simulink model "HEVModel"  (R2021a)
settings: Solver=ode4  StartTime=0  StopTime=tEnd  FixedStep=dt  RelTol=1e-3
values from neighbouring files (symbols this model uses):
  accessoryLoad = 600    [main.m]
  Af = 1.00    (= 1)    [main.m]
  batteryCapacity = 50    [main.m]
  batteryResistance = 0.0461    [main.m]
  C = 400    [main.m]
  Cd = 0.576    [main.m]
  Crr = 0.01    [main.m]
  cycleNum = 2    [main.m]
  EffTableEff = [.75 .85 .89 .95 .96 .97 .98 .99 .99]    [main.m]
  EffTableSpeed = [0 5 10 15 25 35 45 55 65]    [main.m]
  etaGenGR = 0.93    [main.m]
  g = 9.81    [main.m]
  genMotorData = load(GENERATOR_MOTOR_DATA_NAME)    [main.m]
  GRd = 9.843    [main.m]
  GRgen = 1.4    [main.m]
  initialGasVolume = 5    [main.m]
  k_gal2kWh = 32.3    [main.m]
  k_hr2s = 3600    [main.m]
  k_J2gal = 1/3600000/32.3    (= 8.59993120055e-09)    [main.m]
  k_kW2W = 1000    [main.m]
  k_kWh2J = 3.6*10^6    (= 3600000)    [main.m]
  k_m2mi = 0.000621371    [main.m]
  k_m32gal = 264.172    [main.m]
  k_rpm2rps = 2*pi()/60    [main.m]
  k_rps2rpm = 60/(2*pi)    (= 9.54929658551)    [main.m]
  k_s2h = 1/3600    (= 0.000277777777778)    [main.m]
  k_W2kW = 1/1000    (= 0.001)    [main.m]
  kc = 0.513    [main.m]
  Kd = 0    [main.m]
  Ki = 0.1    [main.m]
  ki = 0.0773    [main.m]
  Kp = 200    [main.m]
  kw = 0.0000064    (= 6.4e-06)    [main.m]
  m = 1965    [main.m]
  motorMaxPower = 310000    [main.m]
  motorMaxSpeed = 18000    [main.m]
  motorMaxTorque = 600    [main.m]
  openCircuitVoltage = 420    [main.m]
  pBrakeMax = 4*TbrakeMax / (mu_k*pi()* cylinderBore^2 *meanPadRadius*numPads)    [main.m]
  r = 0.290    (= 0.29)    [main.m]
  rho = 1.20    (= 1.2)    [main.m]
  SOCi = 90    [main.m]
  theta = 0    [main.m]
  v0 = 0    [main.m]
  x0 = 0    [main.m]
libraries: autolibshared x6, fl_lib x5, nesl_utility x5, sdl_lib x1, autolibsharedmappedengines x1
(part 3 of 3)

== system HEVModel/Plant/Genset/Gearbox ==
  Torque In [Nm] : Inport
  Power In [W] : Inport  Port=2
  Engine Speed [rad/s] : Inport  Port=3
  Add : Sum  Inputs=+-
  Bus Creator : BusCreator  Inputs=3
  Gain : Gain  Gain=GRgen
  Gain1 : Gain  Gain=k_W2kW
  Gain2 : Gain  Gain=etaGenGR
  Gain3 : Gain  Gain=1/GRgen
  Product1 : Product
  Torque Out [Nm] : Outport
  Info : Outport  Port=2
  wires:
  Gain2/1 -> [torqueOut], Torque Out [Nm]/1, Product1/1  "Torque Out [Nm]"
  Product1/1 -> Add/2  "Gearbox Power Out [W]"
  Engine Speed [rad/s]/1 -> Gain3/1
  Gain/1 -> Gain2/1
  Power In [W]/1 -> Add/1
  Add/1 -> Gain1/1  "Gearbox Power Loss [W]"
  Torque In [Nm]/1 -> [torqueIn], Gain/1
  Gain1/1 -> Bus Creator/1  "powerLoss"
  [torqueIn] -> Bus Creator/2  "torqueIn"
  [torqueOut] -> Bus Creator/3  "torqueOut"
  Bus Creator/1 -> Info/1  "gearbox"
  Gain3/1 -> Product1/2

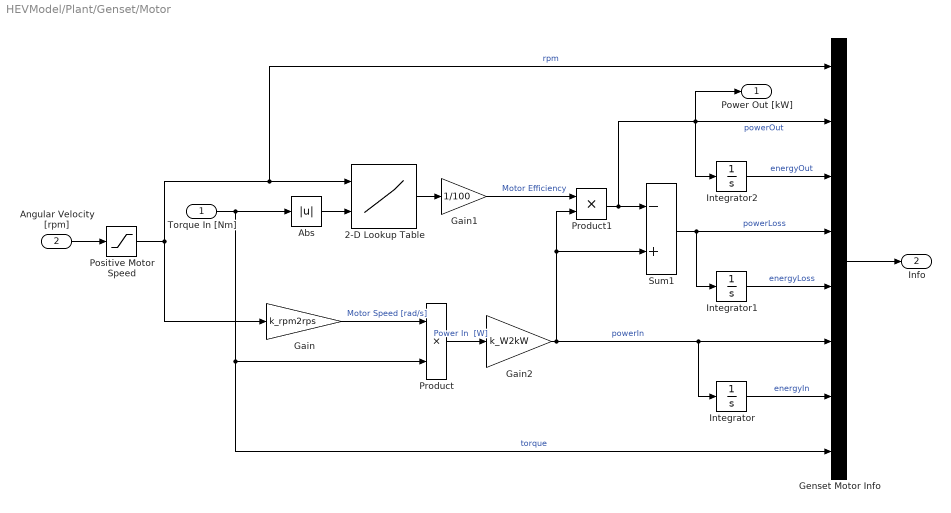
== system HEVModel/Plant/Genset/Motor ==
  Torque In [Nm] : Inport
  Angular Velocity [rpm] : Inport  Port=2
  2-D Lookup Table : Lookup_n-D  BreakpointsForDimension1=genMotorData.w_eff_bp  BreakpointsForDimension2=genMotorData.T_eff_bp  Table=genMotorData.efficiency_table  InternalRulePriority=Speed  RndMeth=Simplest  InputSameDT=on
      settings: InputPortMap=u0,u1
  Abs : Abs
  Gain : Gain  Gain=k_rpm2rps
  Gain1 : Gain  Gain=1/100
  Gain2 : Gain  Gain=k_W2kW
  Genset Motor Info : BusCreator  Inputs=8
  Integrator : Integrator
  Integrator1 : Integrator
  Integrator2 : Integrator
  Positive Motor Speed : Saturate  UpperLimit=inf  LowerLimit=0
  Product : Product
  Product1 : Product
  Sum1 : Sum  Inputs=-+
  Power Out [kW] : Outport
  Info : Outport  Port=2
  wires:
  Angular Velocity [rpm]/1 -> Positive Motor Speed/1
  Gain/1 -> Product/1  "Motor Speed [rad/s]"
  Positive Motor Speed/1 -> Genset Motor Info/1, 2-D Lookup Table/1, Gain/1  "rpm"
  Gain1/1 -> Product1/1  "Motor Efficiency"
  Product1/1 -> Sum1/1, Power Out [kW]/1, Genset Motor Info/2, Integrator2/1  "powerOut"
  Integrator2/1 -> Genset Motor Info/3  "energyOut"
  Sum1/1 -> Genset Motor Info/4, Integrator1/1  "powerLoss"
  2-D Lookup Table/1 -> Gain1/1
  Abs/1 -> 2-D Lookup Table/2
  Integrator1/1 -> Genset Motor Info/5  "energyLoss"
  Integrator/1 -> Genset Motor Info/7  "energyIn"
  Torque In [Nm]/1 -> Abs/1, Genset Motor Info/8, Product/2  "torque"
  Gain2/1 -> Integrator/1, Genset Motor Info/6, Sum1/2, Product1/2  "powerIn"
  Genset Motor Info/1 -> Info/1
  Product/1 -> Gain2/1  "Power In  [W]"

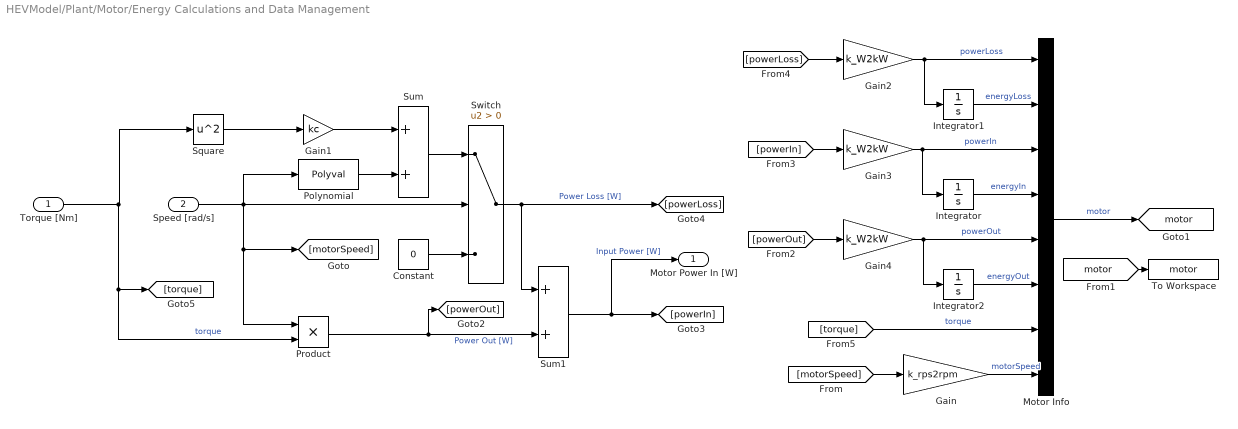
== system HEVModel/Plant/Motor/Energy Calculations and Data Management ==
  Torque [Nm] : Inport
  Speed [rad/s] : Inport  Port=2
  Constant : Constant  Value=0
  Gain : Gain  Gain=k_rps2rpm
  Gain1 : Gain  Gain=kc
  Gain2 : Gain  Gain=k_W2kW
  Gain3 : Gain  Gain=k_W2kW
  Gain4 : Gain  Gain=k_W2kW
  Integrator : Integrator
  Integrator1 : Integrator
  Integrator2 : Integrator
  Motor Info : BusCreator  Inputs=8
  Polynomial : Polyval  Coefs=[kw , 0 ki, C]
  Product : Product
  Square : Math  Operator=square  SaturateOnIntegerOverflow=on
  Sum : Sum
  Sum1 : Sum
  Switch : Switch  Criteria=u2 > Threshold
  To Workspace : ToWorkspace  VariableName=motor  SaveFormat=Timeseries  SampleTime=-1
  Motor Power In [W] : Outport
  tag scope: motor=global
  wires:
  Motor Info/1 -> [motor]  "motor"
  Product/1 -> [powerOut], Sum1/2  "Power Out [W]"
  Speed [rad/s]/1 -> Polynomial/1, Product/1, [motorSpeed], Switch/2
  Constant/1 -> Switch/3
  Polynomial/1 -> Sum/2
  Sum/1 -> Switch/1
  Gain1/1 -> Sum/1
  Switch/1 -> Sum1/1, [powerLoss]  "Power Loss [W]"
  Sum1/1 -> Motor Power In [W]/1, [powerIn]  "Input Power [W]"
  Torque [Nm]/1 -> Square/1, Product/2, [torque]  "torque"
  Square/1 -> Gain1/1
  Integrator/1 -> Motor Info/4  "energyIn"
  Integrator2/1 -> Motor Info/6  "energyOut"
  Integrator1/1 -> Motor Info/2  "energyLoss"
  [motorSpeed] -> Gain/1
  Gain/1 -> Motor Info/8  "motorSpeed"
  [motor] -> To Workspace/1
  Gain4/1 -> Integrator2/1, Motor Info/5  "powerOut"
  Gain3/1 -> Motor Info/3, Integrator/1  "powerIn"
  Gain2/1 -> Motor Info/1, Integrator1/1  "powerLoss"
  [torque] -> Motor Info/7  "torque"
  [powerLoss] -> Gain2/1
  [powerIn] -> Gain3/1
  [powerOut] -> Gain4/1

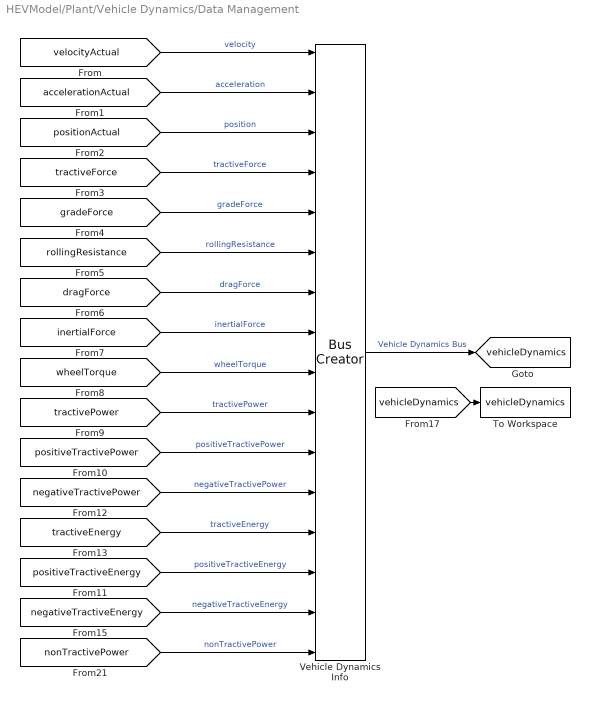
== system HEVModel/Plant/Vehicle Dynamics/Data Management ==
  To Workspace : ToWorkspace  VariableName=vehicleDynamics  SaveFormat=Timeseries  SampleTime=-1
  Vehicle Dynamics Info : BusCreator  Inputs=16
  tag scope: vehicleDynamics=global
  wires:
  [velocityActual] -> Vehicle Dynamics Info/1  "velocity"
  [wheelTorque] -> Vehicle Dynamics Info/9  "wheelTorque"
  [tractiveForce] -> Vehicle Dynamics Info/4  "tractiveForce"
  [negativeTractivePower] -> Vehicle Dynamics Info/12  "negativeTractivePower"
  [accelerationActual] -> Vehicle Dynamics Info/2  "acceleration"
  [vehicleDynamics] -> To Workspace/1
  [gradeForce] -> Vehicle Dynamics Info/5  "gradeForce"
  [positiveTractivePower] -> Vehicle Dynamics Info/11  "positiveTractivePower"
  [positiveTractiveEnergy] -> Vehicle Dynamics Info/14  "positiveTractiveEnergy"
  [rollingResistance] -> Vehicle Dynamics Info/6  "rollingResistance"
  [inertialForce] -> Vehicle Dynamics Info/8  "inertialForce"
  [positionActual] -> Vehicle Dynamics Info/3  "position"
  [tractivePower] -> Vehicle Dynamics Info/10  "tractivePower"
  [negativeTractiveEnergy] -> Vehicle Dynamics Info/15  "negativeTractiveEnergy"
  [tractiveEnergy] -> Vehicle Dynamics Info/13  "tractiveEnergy"
  [dragForce] -> Vehicle Dynamics Info/7  "dragForce"
  [nonTractivePower] -> Vehicle Dynamics Info/16  "nonTractivePower"
  Vehicle Dynamics Info/1 -> [vehicleDynamics]  "Vehicle Dynamics Bus"

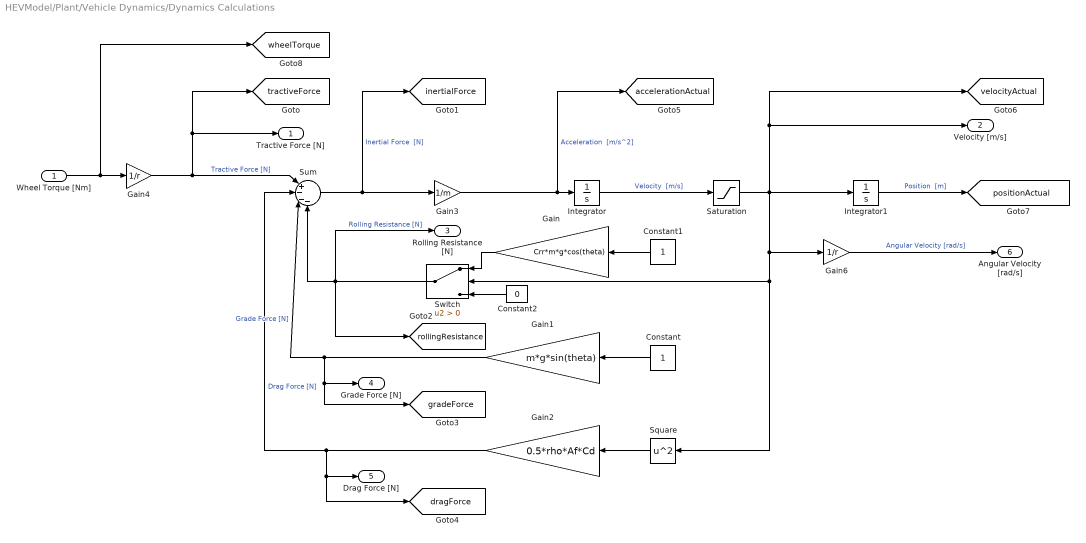
== system HEVModel/Plant/Vehicle Dynamics/Dynamics Calculations ==
  Wheel Torque [Nm] : Inport
  Constant : Constant
  Constant1 : Constant
  Constant2 : Constant  Value=0
  Gain : Gain  Gain=Crr*m*g*cos(theta)
  Gain1 : Gain  Gain=m*g*sin(theta)
  Gain2 : Gain  Gain=0.5*rho*Af*Cd
  Gain3 : Gain  Gain=1/m
  Gain4 : Gain  Gain=1/r
  Gain6 : Gain  Gain=1/r
  Integrator : Integrator  InitialCondition=v0
  Integrator1 : Integrator  InitialCondition=x0
  Saturation : Saturate  UpperLimit=inf  LowerLimit=0  LinearizeAsGain=off
  Square : Math  Operator=square  SaturateOnIntegerOverflow=on
  Sum : Sum  Inputs=|+---
  Switch : Switch  Criteria=u2 > Threshold
  Tractive Force [N] : Outport
  Velocity [m/s] : Outport  Port=2
  Rolling Resistance [N] : Outport  Port=3
  Grade Force [N] : Outport  Port=4
  Drag Force [N] : Outport  Port=5
  Angular Velocity [rad/s] : Outport  Port=6
  tag scope: accelerationActual=global, dragForce=global, gradeForce=global, inertialForce=global, positionActual=global, rollingResistance=global, tractiveForce=global, velocityActual=global, wheelTorque=global
  wires:
  Gain1/1 -> Grade Force [N]/1, [gradeForce], Sum/3  "Grade Force [N]"
  Gain4/1 -> Tractive Force [N]/1, [tractiveForce], Sum/1  "Tractive Force [N]"
  Constant/1 -> Gain1/1
  Switch/1 -> Sum/4, [rollingResistance], Rolling Resistance [N]/1  "Rolling Resistance [N]"
  Integrator/1 -> Saturation/1  "Velocity  [m/s]"
  Integrator1/1 -> [positionActual]  "Position  [m]"
  Sum/1 -> [inertialForce], Gain3/1  "Inertial Force  [N]"
  Constant1/1 -> Gain/1
  Gain3/1 -> [accelerationActual], Integrator/1  "Acceleration  [m/s^2]"
  Gain2/1 -> Drag Force [N]/1, [dragForce], Sum/2  "Drag Force [N]"
  Wheel Torque [Nm]/1 -> [wheelTorque], Gain4/1
  Square/1 -> Gain2/1
  Saturation/1 -> Gain6/1, Square/1, Switch/2, Velocity [m/s]/1, [velocityActual], Integrator1/1
  Gain/1 -> Switch/1
  Constant2/1 -> Switch/3
  Gain6/1 -> Angular Velocity [rad/s]/1  "Angular Velocity [rad/s]"

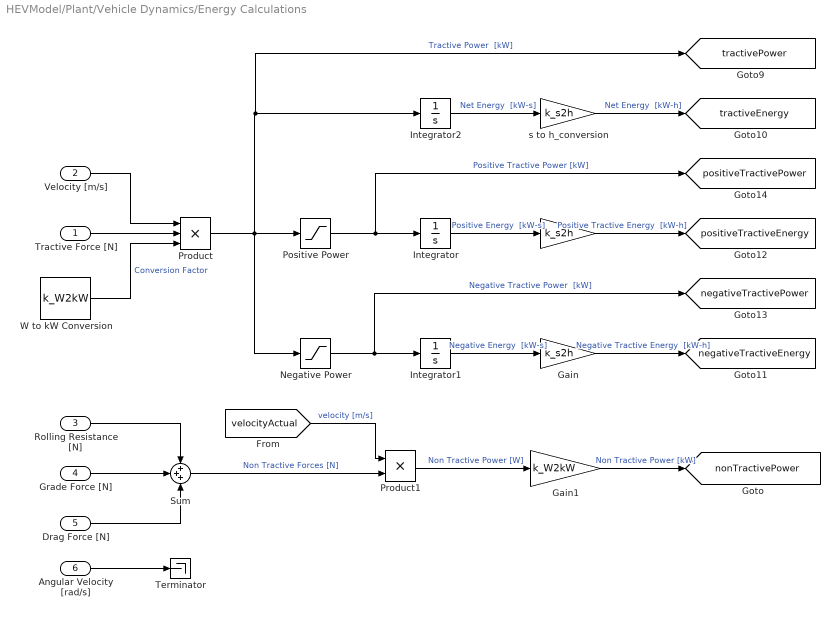
== system HEVModel/Plant/Vehicle Dynamics/Energy Calculations ==
  Tractive Force [N] : Inport
  Velocity [m/s] : Inport  Port=2
  Rolling Resistance [N] : Inport  Port=3
  Grade Force [N] : Inport  Port=4
  Drag Force [N] : Inport  Port=5
  Angular Velocity [rad/s] : Inport  Port=6
  " " : Gain  Gain=k_s2h
  Gain : Gain  Gain=k_s2h
  Gain1 : Gain  Gain=k_W2kW
  Integrator : Integrator
  Integrator1 : Integrator
  Integrator2 : Integrator
  Negative Power : Saturate  UpperLimit=0  LowerLimit=-inf
  Positive Power : Saturate  UpperLimit=inf  LowerLimit=0
  Product : Product  Inputs=3
  Product1 : Product
  Sum : Sum  Inputs=+++
  Terminator : Terminator
  W to kW Conversion : Constant  Value=k_W2kW
  s to h_conversion : Gain  Gain=k_s2h
  tag scope: negativeTractiveEnergy=global, negativeTractivePower=global, nonTractivePower=global, positiveTractiveEnergy=global, positiveTractivePower=global, tractiveEnergy=global, tractivePower=global
  wires:
  s to h_conversion/1 -> [tractiveEnergy]  "Net Energy  [kW-h]"
  " "/1 -> [positiveTractiveEnergy]  "Positive Tractive Energy  [kW-h]"
  Gain/1 -> [negativeTractiveEnergy]  "Negative Tractive Energy  [kW-h]"
  Integrator1/1 -> Gain/1  "Negative Energy  [kW-s]"
  Integrator/1 -> " "/1  "Positive Energy  [kW-s]"
  Negative Power/1 -> [negativeTractivePower], Integrator1/1  "Negative Tractive Power  [kW]"
  Integrator2/1 -> s to h_conversion/1  "Net Energy  [kW-s]"
  Positive Power/1 -> [positiveTractivePower], Integrator/1  "Positive Tractive Power [kW]"
  W to kW Conversion/1 -> Product/3  "Conversion Factor"
  Product/1 -> Negative Power/1, [tractivePower], Integrator2/1, Positive Power/1  "Tractive Power  [kW]"
  Velocity [m/s]/1 -> Product/1
  Tractive Force [N]/1 -> Product/2
  Drag Force [N]/1 -> Sum/3
  Grade Force [N]/1 -> Sum/2
  Rolling Resistance [N]/1 -> Sum/1
  Sum/1 -> Product1/2  "Non Tractive Forces [N]"
  [velocityActual] -> Product1/1  "velocity [m/s]"
  Product1/1 -> Gain1/1  "Non Tractive Power [W]"
  Gain1/1 -> [nonTractivePower]  "Non Tractive Power [kW]"
  Angular Velocity [rad/s]/1 -> Terminator/1

== stateflow chart HEVModel/Plant/Thermostatic Hybrid Supervisory Controller /Chart ==
  state second
    entry:
    EngineTorque = 65;
    MotorSpeed = 800;
  state first
    entry:
    EngineTorque = 0;
    MotorSpeed = 0;
  (default) -> first
  first -> second : [FuelTankVolume > 0.2 && SOC < 85]
  second -> first : [FuelTankVolume < 0.2 || SOC > 90]
  data: SOC input; FuelTankVolume input; EngineTorque output; MotorSpeed output
